simulink model "compliance_adjusting_PLUS_energy_aware_controller"  (R2020b)
settings: Solver=VariableStepAuto  StartTime=0.0  StopTime=42  RelTol=1e-3
values from neighbouring files (symbols this model uses):
  alpha = 0.001    [compliance_PLUS_energy_setup.m]    (also in compliance_adjusting_setup.m = 2; hyperbole_test.m = 1000)
  b0 = 2 * sqrt(k0 * m_R)    [compliance_PLUS_energy_setup.m]    (also in compliance_adjusting_setup.m = 2; energy_aware_setup.m = 20; optim_criteria.m = 0.2; plot_meshes.m = 0.2)
  C_max = 10    [compliance_PLUS_energy_setup.m]    (also in compliance_adjusting_setup.m = 0.2)
  E_max = 1    [compliance_PLUS_energy_setup.m]    (also in energy_aware_setup.m = 0.7; optim_criteria.m = 0.5; plot_meshes.m = 0.5; setup.m)
  F_cmax = 5    [compliance_PLUS_energy_setup.m]    (also in compliance_adjusting_setup.m)
  k0 = 20    [compliance_PLUS_energy_setup.m]    (also in compliance_adjusting_setup.m = 10; energy_aware_setup.m = 100; optim_criteria.m = 1; plot_meshes.m = 1)
  km = 100    [compliance_PLUS_energy_setup.m]    (also in compliance_adjusting_setup.m; energy_aware_setup.m; setup.m)
  m_R = 1    [compliance_PLUS_energy_setup.m]    (also in compliance_adjusting_setup.m; energy_aware_setup.m; setup.m)
  P_max = 1    [compliance_PLUS_energy_setup.m]    (also in energy_aware_setup.m = 0.2; optim_criteria.m = 0.5; plot_meshes.m = 0.5; setup.m = 0.1)
  s0 = 5    [compliance_PLUS_energy_setup.m]    (also in energy_aware_setup.m; setup.m)
  sigma = 0    [compliance_PLUS_energy_setup.m]    (also in compliance_adjusting_setup.m)
  T = 1/30    (= 0.0333333333333)    [compliance_PLUS_energy_setup.m]    (also in compliance_adjusting_setup.m)
  t_collision = 20    [compliance_PLUS_energy_setup.m]    (also in compliance_adjusting_setup.m; energy_aware_setup.m; setup.m)
  t_init = 2    [compliance_PLUS_energy_setup.m]    (also in compliance_adjusting_setup.m; energy_aware_setup.m; setup.m)
  x_O = 0.5    [compliance_PLUS_energy_setup.m]    (also in compliance_adjusting_setup.m; energy_aware_setup.m; setup.m)
  x_O2 = -2    [compliance_PLUS_energy_setup.m]    (also in compliance_adjusting_setup.m)
  x_R = 0    [compliance_PLUS_energy_setup.m]    (also in compliance_adjusting_setup.m; energy_aware_setup.m; setup.m)
libraries: neural x1
settings Model: Creator=kika  LastModifiedBy=kika

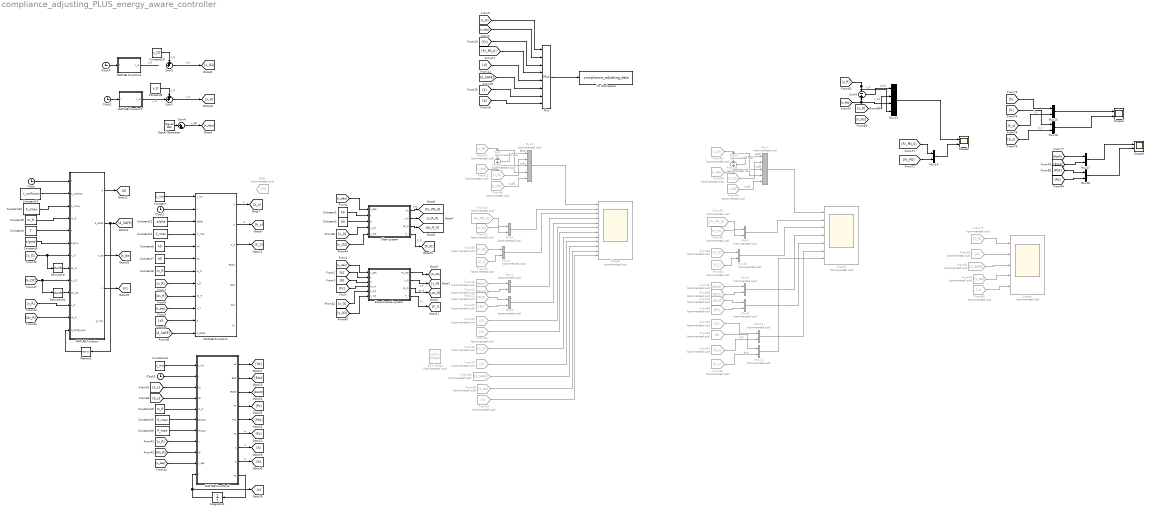
== system compliance_adjusting_PLUS_energy_aware_controller ==
  Clear system : Subsystem
  Clock{,1..4} (5 alike) : Clock
  Constant : Constant  Value=t_init
  Constant1 : Constant  Value=k0
  Constant10 : Constant  Value=F_cmax
  Constant11 : Constant  Value=C_max
  Constant12 : Constant  Value=alpha
  Constant13 : Constant  Value=t_collision
  Constant14 : Constant  Value=t_init
  Constant15 : Constant  Value=E_max
  Constant16 : Constant  Value=P_max
  Constant19 : Constant  Value=m_R
  Constant2 : Constant  Value=b0
  Constant20 : Constant  Value=x_O2
  Constant3 : Constant  Value=sigma
  Constant4 : Constant  Value=T
  Constant5 : Constant  Value=x_O
  Constant6 : Constant  Value=k0
  Constant7 : Constant  Value=b0
  Constant8 : Constant  Value=m_R
  Constant9 : Constant  Value=m_R
  Derivative : Derivative
  Derivative1 : Derivative
  Experimental system : Subsystem
  From10 : From  Commented=on  GotoTag=x_R
  From11 : From  Commented=on  GotoTag=x_des
  From12 : From  Commented=on  GotoTag=Fc_PD
  From13 : From  Commented=on  GotoTag=C_S
  From16 : From  Commented=on  GotoTag=Etot0
  From17 : From  Commented=on  GotoTag=k
  From18 : From  Commented=on  GotoTag=b
  From19 : From  Commented=on  GotoTag=Fc_PD_0
  From21 : From  Commented=on  GotoTag=Etot
  From22 : From  Commented=on  GotoTag=Pc0
  From23 : From  Commented=on  GotoTag=Pc
  From24 : From  Commented=on  GotoTag=x_O
  From28 : From  Commented=on  GotoTag=t_da
  From29 : From  Commented=on  GotoTag=n
  From37 : From  Commented=on  GotoTag=d
  From38 : From  Commented=on  GotoTag=d_SAFE
  From39 : From  Commented=on  GotoTag=F_I0
  From40 : From  Commented=on  GotoTag=F_I
  From46 : From  Commented=on  GotoTag=x_O2
  From48 : From  Commented=on  GotoTag=x_R
  From49 : From  Commented=on  GotoTag=x_des
  From50 : From  Commented=on  GotoTag=Fc_PD
  From52 : From  Commented=on  GotoTag=Etot0
  From53 : From  Commented=on  GotoTag=k
  From54 : From  Commented=on  GotoTag=b
  From55 : From  Commented=on  GotoTag=Fc_PD_0
  From56 : From  Commented=on  GotoTag=Etot
  From57 : From  Commented=on  GotoTag=Pc0
  From58 : From  Commented=on  GotoTag=Pc
  From59 : From  Commented=on  GotoTag=x_O
  From61 : From  Commented=on  GotoTag=k_s
  From62 : From  Commented=on  GotoTag=b_s
  From64 : From  Commented=on  GotoTag=F_I0
  From65 : From  Commented=on  GotoTag=F_I
  From66 : From  Commented=on  GotoTag=x_O2
  From70 : From  Commented=on  GotoTag=C_S
  From79 : From  Commented=on  GotoTag=t_da
  From80 : From  Commented=on  GotoTag=n
  From81 : From  Commented=on  GotoTag=d
  From82 : From  Commented=on  GotoTag=d_SAFE
  Goto : Goto  Commented=on  GotoTag=Fc
  Integrator4 : Integrator  InitialCondition=s0
  MATLAB Function : MATLAB Function  TreatAsAtomicUnit=on
  MATLAB Function1 : MATLAB Function  TreatAsAtomicUnit=on
  MATLAB Function2 : MATLAB Function  TreatAsAtomicUnit=on
  MATLAB Function3 : MATLAB Function  TreatAsAtomicUnit=on
  MATLAB Function4 : MATLAB Function  TreatAsAtomicUnit=on
  Memory : Memory
  Mux : Mux  Inputs=8
  Mux{1,3..6,8..12} (10 alike) : Mux  Commented=on  Inputs=2
  Mux13 : Mux
  Mux{14..18} (5 alike) : Mux  Inputs=2
  Mux2 : Mux  Commented=on  Inputs=5
  Mux7 : Mux  Commented=on  Inputs=5
  Scope : Scope  Commented=on  NumInputPorts=12
  Scope1 : Scope  Commented=on  NumInputPorts=7
  Scope2 : Scope  Commented=on  NumInputPorts=5
  Scope3 : Scope  NumInputPorts=2
  Scope4 : Scope  NumInputPorts=2
  Scope5 : Scope  NumInputPorts=2
  Signal Generator : SignalGenerator  Frequency=0.5  Units=rad/sec
  Sum : Sum  Commented=on  Inputs=-+
  Sum1 : Sum  Inputs=++|
  Sum2 : Sum  Inputs=++|
  Sum3 : Sum  Commented=on  Inputs=-+
  Sum4 : Sum  Inputs=|++
  Sum5 : Sum  Inputs=-+
  To Workspace : ToWorkspace  VariableName=compliance_adjusting_data  SaveFormat=Timeseries  SampleTime=-1
  X(2Y) Graph : neural/Control Systems/X(2Y)  Graph  Commented=on  xmin=0  xmax=5  ymin=21  ymax=22  st=-1
      settings: SourceProductBaseCode=NN
  wires:
  Constant7/1 -> MATLAB Function1/6(b0)
  MATLAB Function1/1(k) -> [k_s]  "k"
  Constant8/1 -> MATLAB Function1/7(m_R)
  Constant6/1 -> MATLAB Function1/5(k0)
  Clock2/1 -> MATLAB Function1/2(t)
  MATLAB Function1/2(b) -> [b_s]  "b"
  Signal Generator/1 -> Sum4/1
  Constant/1 -> MATLAB Function1/1(t_init)
  [Fc] -> Experimental system/4(Fc_in)
  [x_des] -> Experimental system/1(x_des)
  Experimental system/2(x_R) -> [x_R]  "x_R"
  Experimental system/3(dx_R) -> [dx_R]  "dx_R"
  Experimental system/1(Fc_PD) -> [Fc_PD]
  Clear system/1(Fc) -> [Fc_PD_0]  "Fc0"
  Clear system/2(x_R) -> [x_R_0]
  Clear system/3(dx_R) -> [dx_R_0]
  [k] -> Experimental system/2(k)
  [b] -> Experimental system/3(b)
  [x_des] -> Clear system/1(x_des)
  Constant1/1 -> Clear system/2(k)
  Constant2/1 -> Clear system/3(b)
  [dx_R] -> MATLAB Function1/9(dx_R)
  [x_R] -> MATLAB Function1/8(x_R)
  Sum4/1 -> [x_des]  "x_des"
  [x_des] -> MATLAB Function1/10(x_V)
  From10/1 -> Mux2/4, Sum/1
  From11/1 -> Mux2/3, Sum/2
  Mux2/1 -> Scope/1
  From12/1 -> Mux4/2
  From17/1 -> Scope/6
  From18/1 -> Scope/7
  From19/1 -> Mux4/1
  Mux4/1 -> Scope/2
  Sum/1 -> Mux2/1  "error"
  Mux/1 -> To Workspace/1
  [x_O] -> Experimental system/5(x_O1)
  [x_O] -> Clear system/4(x_O1)
  [x_O] -> Derivative/1, MATLAB Function/7(x_O)
  [x_R] -> MATLAB Function/11(x_R)
  [dx_R] -> MATLAB Function/12(dx_R)
  Derivative/1 -> MATLAB Function/8(dx_O)
  Constant3/1 -> MATLAB Function/6(sigma)
  Constant4/1 -> MATLAB Function/5(T)
  Constant9/1 -> MATLAB Function/4(m_R)
  Constant10/1 -> MATLAB Function/3(F_cmax)
  Constant11/1 -> MATLAB Function1/4(C_max)
  Constant12/1 -> MATLAB Function1/3(alpha)
  [d_SAFE] -> MATLAB Function1/12(d_SAFE)
  [d] -> MATLAB Function1/11(d)
  MATLAB Function/1(d) -> [d]
  MATLAB Function/2(d_SAFE) -> Memory/1, [d_SAFE]
  Constant13/1 -> MATLAB Function/2(t_collition)
  Clock/1 -> MATLAB Function/1(t)
  MATLAB Function1/3(C_S) -> [C_S]
  From13/1 -> Scope/8
  [d_SAFE] -> Mux/6
  [Fc_PD_0] -> Mux/4
  [d] -> Mux/5
  [k] -> Mux/7
  [b] -> Mux/8
  [Fc] -> Mux/3
  [x_des] -> Mux/2
  [x_R] -> Mux/1
  From37/1 -> Scope/9
  From38/1 -> Scope/10
  Mux1/1 -> Scope/4
  Mux3/1 -> Scope/5
  From16/1 -> Mux1/1
  From21/1 -> Mux1/2
  From22/1 -> Mux3/1
  From23/1 -> Mux3/2
  Constant5/1 -> Sum1/1  "x_O"
  From24/1 -> Mux2/2  "x_O1"
  Sum1/1 -> [x_O]  "x_O"
  MATLAB Function2/1(x_O) -> Sum1/2  "x_O"
  Clock1/1 -> MATLAB Function2/1(t)
  Memory/1 -> MATLAB Function/13(d_SAFE_prev)
  MATLAB Function/3(t_da) -> [t_da]
  MATLAB Function/4(n) -> [n]
  From28/1 -> Scope/11
  From29/1 -> Scope/12
  Clear system/4(F_I) -> [F_I0]  "F_I0"
  Experimental system/4(F_I) -> [F_I]  "F_I"
  From39/1 -> Mux5/1
  From40/1 -> Mux5/2
  Mux5/1 -> Scope/3
  Integrator4/1 -> MATLAB Function3/11(s), [s]
  [b_s] -> MATLAB Function3/4(b0)
  Constant15/1 -> MATLAB Function3/6(Emax0)
  Constant19/1 -> MATLAB Function3/5(m_R)
  MATLAB Function3/7(k) -> [k]  "k"
  Clock3/1 -> MATLAB Function3/2(t)
  Constant14/1 -> MATLAB Function3/1(t_init)
  MATLAB Function3/5(Pc0) -> [Pc0]
  MATLAB Function3/3(Etot0) -> [Etot0]
  MATLAB Function3/8(b) -> [b]  "b"
  [x_R] -> MATLAB Function3/8(x)
  [k_s] -> MATLAB Function3/3(k0)
  [x_des] -> MATLAB Function3/10(x_des)
  MATLAB Function3/6(Fc) -> [Fc]  "Fc"
  [dx_R] -> MATLAB Function3/9(dx)
  MATLAB Function3/2(Etot) -> [Etot]
  MATLAB Function3/9(ds) -> Integrator4/1
  Constant16/1 -> MATLAB Function3/7(Pmax0)
  MATLAB Function3/1(Hs) -> [Hs]
  MATLAB Function3/4(Pc) -> [Pc]
  [x_O2] -> Clear system/5(x_O2)
  [x_O2] -> Experimental system/6(x_O2)
  Constant20/1 -> Sum2/1  "x_O"
  MATLAB Function4/1(x_O) -> ?  "x_O"
  Sum2/1 -> [x_O2]  "x_O"
  Clock4/1 -> MATLAB Function4/1(t)
  From46/1 -> Mux2/5  "x_O2"
  [x_O2] -> Derivative1/1, MATLAB Function/9(x_O2)
  Derivative1/1 -> MATLAB Function/10(dx_O2)
  From52/1 -> Mux6/1
  Mux8/1 -> Scope1/5
  Mux9/1 -> Scope1/2
  Mux7/1 -> Scope1/1
  From58/1 -> Mux8/2
  Sum3/1 -> Mux7/1  "error"
  Mux10/1 -> Scope1/3
  From56/1 -> Mux6/2
  From55/1 -> Mux9/1
  From64/1 -> Mux10/1
  From66/1 -> Mux7/5  "x_O2"
  From57/1 -> Mux8/1
  From48/1 -> Mux7/4, Sum3/1
  From65/1 -> Mux10/2
  Mux11/1 -> Scope1/6
  From50/1 -> Mux9/2
  Mux6/1 -> Scope1/4
  From59/1 -> Mux7/2  "x_O1"
  From49/1 -> Mux7/3, Sum3/2
  Mux12/1 -> Scope1/7
  From70/1 -> Scope2/1
  From81/1 -> Scope2/2
  From82/1 -> Scope2/3
  From79/1 -> Scope2/4
  From80/1 -> Scope2/5
  From61/1 -> Mux11/2  "k_s"
  From62/1 -> Mux12/2  "b_s"
  From54/1 -> Mux12/1
  From53/1 -> Mux11/1
  [x_O] -> Mux13/2  "x_O1"
  [x_R] -> Mux13/4, Sum5/1  "x_R"
  Mux13/1 -> Scope3/1
  Sum5/1 -> Mux13/1  "error"
  [x_des] -> Mux13/3, Sum5/2
  [Fc_PD_0] -> Mux14/1
  Mux14/1 -> Scope3/2
  [Fc_PD] -> Mux14/2
  Mux16/1 -> Scope4/2
  [k_s] -> Mux15/2  "k_s"
  [b] -> Mux16/1
  [k] -> Mux15/1
  [b_s] -> Mux16/2  "b_s"
  Mux15/1 -> Scope4/1
  Mux18/1 -> Scope5/2
  [Pc] -> Mux18/2
  Mux17/1 -> Scope5/1
  [Etot0] -> Mux17/1
  [Etot] -> Mux17/2
  [Pc0] -> Mux18/1

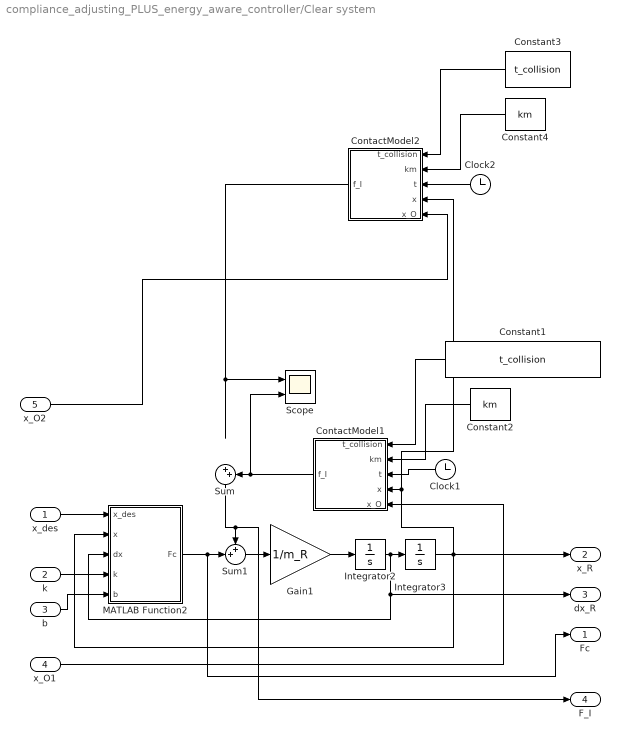
== system compliance_adjusting_PLUS_energy_aware_controller/Clear system ==
  x_des : Inport
  k : Inport  Port=2
  b : Inport  Port=3
  x_O1 : Inport  Port=4
  x_O2 : Inport  Port=5
  Clock1 : Clock
  Clock2 : Clock
  Constant1 : Constant  Value=t_collision
  Constant2 : Constant  Value=km
  Constant3 : Constant  Value=t_collision
  Constant4 : Constant  Value=km
  ContactModel1 : MATLAB Function  TreatAsAtomicUnit=on
  ContactModel2 : MATLAB Function  TreatAsAtomicUnit=on
  Gain1 : Gain  Gain=1/m_R
  Integrator2 : Integrator
  Integrator3 : Integrator  InitialCondition=x_R
  MATLAB Function2 : MATLAB Function  TreatAsAtomicUnit=on
  Scope : Scope  NumInputPorts=2
  Sum : Sum  Inputs=|++
  Sum1 : Sum  Inputs=++|
  Fc : Outport
  x_R : Outport  Port=2
  dx_R : Outport  Port=3
  F_I : Outport  Port=4
  wires:
  k/1 -> MATLAB Function2/4(k)
  ContactModel1/1(f_I) -> Scope/2, Sum/2
  Clock1/1 -> ContactModel1/3(t)
  x_des/1 -> MATLAB Function2/1(x_des)
  b/1 -> MATLAB Function2/5(b)
  Sum1/1 -> Gain1/1
  x_O1/1 -> ContactModel1/5(x_O)
  Gain1/1 -> Integrator2/1
  MATLAB Function2/1(Fc) -> Fc/1, Sum1/2
  Integrator2/1 -> dx_R/1, MATLAB Function2/3(dx), Integrator3/1
  Constant1/1 -> ContactModel1/1(t_collision)
  Constant2/1 -> ContactModel1/2(km)
  Constant3/1 -> ContactModel2/1(t_collision)
  Integrator3/1 -> x_R/1, ContactModel2/4(x), ContactModel1/4(x), MATLAB Function2/2(x)
  x_O2/1 -> ContactModel2/5(x_O)
  Constant4/1 -> ContactModel2/2(km)
  Clock2/1 -> ContactModel2/3(t)
  Sum/1 -> F_I/1, Sum1/1
  ContactModel2/1(f_I) -> Scope/1

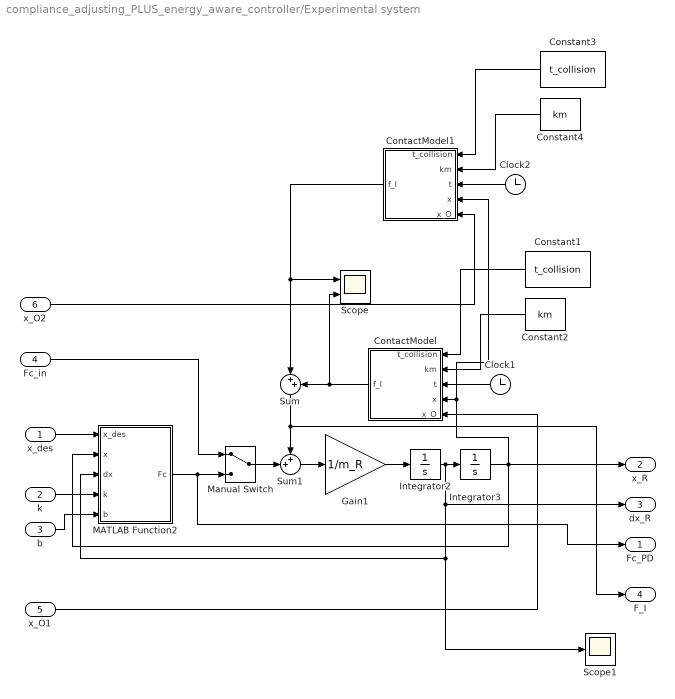
== system compliance_adjusting_PLUS_energy_aware_controller/Experimental system ==
  x_des : Inport
  k : Inport  Port=2
  b : Inport  Port=3
  Fc_in : Inport  Port=4
  x_O1 : Inport  Port=5
  x_O2 : Inport  Port=6
  Clock1 : Clock
  Clock2 : Clock
  Constant1 : Constant  Value=t_collision
  Constant2 : Constant  Value=km
  Constant3 : Constant  Value=t_collision
  Constant4 : Constant  Value=km
  ContactModel : MATLAB Function  TreatAsAtomicUnit=on
  ContactModel1 : MATLAB Function  TreatAsAtomicUnit=on
  Gain1 : Gain  Gain=1/m_R
  Integrator2 : Integrator
  Integrator3 : Integrator  InitialCondition=x_R
  MATLAB Function2 : MATLAB Function  TreatAsAtomicUnit=on
  Manual Switch : ManualSwitch
  Scope : Scope  NumInputPorts=2
  Scope1 : Scope
  Sum : Sum  Inputs=|++
  Sum1 : Sum  Inputs=++|
  Fc_PD : Outport
  x_R : Outport  Port=2
  dx_R : Outport  Port=3
  F_I : Outport  Port=4
  wires:
  k/1 -> MATLAB Function2/4(k)
  ContactModel/1(f_I) -> Scope/2, Sum/2
  Clock1/1 -> ContactModel/3(t)
  Integrator3/1 -> x_R/1, ContactModel1/4(x), ContactModel/4(x), MATLAB Function2/2(x)
  x_des/1 -> MATLAB Function2/1(x_des)
  b/1 -> MATLAB Function2/5(b)
  Sum1/1 -> Gain1/1
  x_O1/1 -> ContactModel/5(x_O)
  Gain1/1 -> Integrator2/1
  MATLAB Function2/1(Fc) -> Manual Switch/2, Fc_PD/1
  Integrator2/1 -> dx_R/1, Scope1/1, MATLAB Function2/3(dx), Integrator3/1
  Constant1/1 -> ContactModel/1(t_collision)
  Constant2/1 -> ContactModel/2(km)
  Fc_in/1 -> Manual Switch/1
  Manual Switch/1 -> Sum1/2
  ContactModel1/1(f_I) -> Sum/1, Scope/1
  Constant4/1 -> ContactModel1/2(km)
  Constant3/1 -> ContactModel1/1(t_collision)
  Clock2/1 -> ContactModel1/3(t)
  x_O2/1 -> ContactModel1/5(x_O)
  Sum/1 -> F_I/1, Sum1/1

== matlab function compliance_adjusting_PLUS_energy_aware_controller/MATLAB Function ==
  data: t input; t_collition input; F_cmax input; m_R input; T input; sigma input; x_O input; dx_O input; x_O2 input; dx_O2 input; d output; x_R input; dx_R input; d_SAFE output; t_da output; n output; a_max output; d_SAFE_prev input
function [d, d_SAFE, t_da, n, a_max] = SENSING(t, t_collition, F_cmax, m_R, T, sigma, x_O, dx_O, x_O2, dx_O2, x_R, dx_R, d_SAFE_prev)

    
    d = 0.1;
    d_SAFE = 0;
    
    
    a_max = F_cmax / m_R;
    t_da1 = abs((dx_R - dx_O) / a_max);
    n1 = ceil(t_da1 / T);
    
    t_da2 = abs((dx_R - dx_O2) / a_max);
    n2 = ceil(t_da2 / T);
    
    t_da = 0;
    d1 = 0;
    d2 = 0;
    d_SAFE = 0;
    n = 0;
    if t > t_collition
        if x_R <= x_O
            d1 = abs(x_R - x_O);
        else
            d1 = 0;
        end
        
        % d_SAFE calculation (deaceleration path length using F_cmax)
        d_SAFE1 = abs(dx_R - dx_O) * n1 * T;
%         d_SAFE = 0.4 * d_SAFE + 0.6 * d_SAFE_prev;
%         d_SAFE = 0.1;
    %     d_SAFE = abs(dx_R - dx_O) * n * T + 3 * sigma;
    
    
        if x_R >= x_O2
            d2 = abs(x_R - x_O2);
        else
            d2 = 0;
        end
        
        % d_SAFE calculation (deaceleration path length using F_cmax)
        d_SAFE2 = abs(dx_R - dx_O2) * n2 * T;
        
        d_SAFE = d_SAFE1;
        d = d1;
        t_da = t_da1;
        n = n1;

        if d1 > d2 && d_SAFE1 > d_SAFE2
            d_SAFE = d_SAFE2;
            d = d2;
            t_da = t_da2;
            n = n2;
        end
        d_SAFE = 0.2;
    end

== matlab function compliance_adjusting_PLUS_energy_aware_controller/MATLAB Function2 ==
  data: t input; x_O output
function x_O = fcn(t)

    offset = -0.3;
    x_O = 1;
    if t > 23 && t < 35
        x_O = sin(0.5 * t + pi);
    end
    if t >= offset + 44.5 && t < offset +46.8
        x_O = 1.5*sin(1.5 * t - pi/6);
    end
    if t > 85
        x_O = 0.2;
    end

== matlab function compliance_adjusting_PLUS_energy_aware_controller/MATLAB Function3 ==
  data: t_init input; t input; k0 input; b0 input; m_R input; Hs output; Emax0 input; Pmax0 input; Etot output; Etot0 output; Pc output; Pc0 output; Fc output; x input; k output; b output; dx input; x_des input; s input; ds output
function [Hs, Etot, Etot0, Pc, Pc0, Fc, k, b, ds] = energy_aware(t_init,t, k0, b0, m_R, Emax0, Pmax0, x, dx, x_des, s)
    
    % initialisation time
    Emax = 1000;
    Pmax = 2000;
    if t > t_init
        Emax = Emax0;
        Pmax = Pmax0;
    end

    e = x_des - x;  % control error
    
    % Kinetic energy
    T = 0.5 * m_R * dx^2;

    % stiffness abjusting using initial Potential energy
    V0 = 0.5 * k0 * e^2;
    Etot0 = T + V0;
    k = k0;
    if Etot0 > Emax
        k = (Emax - T) / (0.5 * e^2);
    end
    if k < 0
        k = 0
    end

    % damping adjusting using new stiffness
    Fs = k * e;
    Fd0 = b0 * dx;
    Fc0 = Fs - Fd0;
    Pc0 = Fc0 * dx;
    b = b0;
    if Pc0 > Pmax
        b = (Fs * dx - Pmax) / dx^2;
    end

    % new control
    Fd = b * dx;
    Fc = Fs - Fd; % control without passivity

    % adjusted total Energy and Power
    V = 0.5 * k * e^2;
    Etot = T + V;
    Pc = Fc * dx;

    % Passivity
    eps = 0.1;
    Hs = 0.5 * s^2;

    u = -Fc * s / sqrt(2 * eps);    % or u = 0;
    if Hs >= eps || Pc < 0
        u = - Fc / s;
    end

    % total contol with passivity
    Fc = -u * s;
    ds = u * dx;

== matlab function compliance_adjusting_PLUS_energy_aware_controller/Experimental system/ContactModel1 ==
  data: t_collision input; km input; t input; f_I output; x input; x_O input
function f_I = fcn(t_collision, km, t, x, x_O)


f_I = 0;

if t > t_collision
    if x < x_O
%     if sign(x * x_O) * (abs(x) - abs(x_O)) > 0
        f_I = km * (x_O - x);
    end
end

== matlab function compliance_adjusting_PLUS_energy_aware_controller/Clear system/ContactModel2 ==
  data: t_collision input; km input; t input; f_I output; x input; x_O input
function f_I = fcn(t_collision, km, t, x, x_O)


f_I = 0;


if t > t_collision
    if x < x_O
        f_I = km * (x_O - x);
    end
end

== matlab function compliance_adjusting_PLUS_energy_aware_controller/MATLAB Function4 ==
  data: t input; x_O output
function x_O = fcn(t)

    x_O = 0;
    if t > 56 && t < 65
        x_O = sin(0.5 * t + pi) + 0.5;
    end
    if t > 71 && t < 85
        x_O = 1.5;
    end
%     if t >= 44.5 && t < 46.8
%         x_O = 3*sin(1.5 * t - pi/4);
%     end

== matlab function compliance_adjusting_PLUS_energy_aware_controller/Experimental system/ContactModel ==
  data: t_collision input; km input; t input; f_I output; x input; x_O input
function f_I = fcn(t_collision, km, t, x, x_O)


f_I = 0;

if t > t_collision
    if x > x_O
%     if sign(x * x_O) * (abs(x) - abs(x_O)) > 0

        f_I = km * (x_O - x);
    end
end

% if t > t_collision
%     if abs(x) - abs(x_O) > 0
%         f_I = km * (abs(x_O) - abs(x));
%     end
% end

== matlab function compliance_adjusting_PLUS_energy_aware_controller/Experimental system/MATLAB Function2 ==
  data: x_des input; Fc output; x input; dx input; k input; b input
function Fc = fcn(x_des, x, dx, k, b)

Fc = k * (x_des - x) - b * dx;

== matlab function compliance_adjusting_PLUS_energy_aware_controller/MATLAB Function1 ==
  data: t_init input; t input; alpha input; C_max input; k0 input; b0 input; m_R input; x_R input; k output; b output; dx_R input; x_V input; d input; d_SAFE input; C_S output; Etot0 output; Etot output; Pc0 output; Pc output
function [k, b, C_S, Etot0, Etot, Pc0, Pc] = compliance(t_init, t, alpha, C_max, k0, b0, m_R, x_R, dx_R, x_V, d, d_SAFE)
    
    k = k0;
    b = b0;
    
    e = x_V - x_R;
    
    Etot0 = 0.5 * m_R * dx_R^2 + 0.5 * k * e^2;
    Pc0 = (k * e - b * dx_R) * dx_R;
    
    C_0 = 1 / k0;
    
    
    D = (C_max * alpha * d)^2 + 4 * C_max * alpha * d_SAFE;
    beta = (-C_max * alpha * d + sqrt(D)) / (2 * C_max);
    gamma = -1 / (alpha * d_SAFE + beta);
        
    C_S = 0;
    if d <= d_SAFE
        C_S = 1 / (alpha * d + beta) + gamma;
    
        k = 1 / (C_0 + C_S);

        % critical damping
        b = 2 * sqrt(k * m_R);
%         
        % Force minimizing
%         b = (k * e * dx_R - 0.1) / dx_R^2;
%        
        if abs(e) < 0.01
            e = sign(e) * 0.01
        end
        if  d > 0.01 && d < 0.2
            b = 1 /d/sign(e);
        end
            
        if b < b0
            b = b0;
        end


% kv = 1;
% E=1;
% k = k0;
% Etot = 0.5 * k * e^2 + 0.5 * kv * (d_SAFE - d)^2 + 0.5 * m_R * dx_R^2;
%         if e == 0
%             e = 0.00001;
%         end
%         k = (e^2)/(2*E - kv * (d_SAFE - d)^2 - m_R * dx_R^2);
%         b = (k * e - kv * (d_SAFE - d)) / dx_R^2;

    
    end
    
    Etot = 0.5 * m_R * dx_R^2 + 0.5 * k * e^2;
    Pc = (k * e - b * dx_R) * dx_R;

== matlab function compliance_adjusting_PLUS_energy_aware_controller/Clear system/MATLAB Function2 ==
  data: x_des input; Fc output; x input; dx input; k input; b input
function Fc = fcn(x_des, x, dx, k, b)

Fc = k * (x_des - x) - b * dx;

== matlab function compliance_adjusting_PLUS_energy_aware_controller/Clear system/ContactModel1 ==
  data: t_collision input; km input; t input; f_I output; x input; x_O input
function f_I = fcn(t_collision, km, t, x, x_O)


f_I = 0;

if t > t_collision
    if x > x_O
        f_I = km * (x_O - x);    
    end
end

% if t > t_collision
%     if abs(x) - abs(x_O) > 0
%         f_I = km * (abs(x_O) - abs(x));
%     end
% end
